simulink model "Copy_of_CM13_2024a_MachE_for_UA_HIL"  (R2024a)
settings: Solver=ode1  StartTime=0.0  StopTime=Inf  FixedStep=0.001  RelTol=1e-3  EnableMultiTasking=on
PreLoadFcn:
  | % if ~length(which('cmcmd')), cmenv; end
PostLoadFcn:
  | if any(exist('dsrtsu_mdlpostloadfcn', 'file') ~= 0), dsrtsu_mdlpostloadfcn('Execute', bdroot); end
InitFcn:
  | , if any(exist('rtifpga_mdlclblib', 'file') ~= 0), rtifpga_mdlclblib('Init', bdroot); end,
  | , if any(exist('dsmpb_private', 'file') ~= 0), dsmpb_private('dsmpb_mdlclblib', 'Init', bdroot); end,
undefined symbols (not defined in the file or in its folder): AccelCmd, ActTqLF_Nm_, ActTqLR_Nm_, ActTqRF_Nm_, ActTqRR_Nm_, BattChargeLimitMaxPwr, BattChargeLimitSocBpts, BattChargeLimitTbl, BattChrgCapcty, BattDischargeLimitSocBpts, BattDischargeLimitTbl, BattDischargeMaxPwr, BattNumCellsParallel, BattNumCellsSeries, BattOpenVoltCapBpts, BattOpenVoltTbl, BattResistSocBpts, BattResistTbl, BattResistTempBpts, BrakeMaxPrs, BrakeMaxTrq, ChassisDistCg2FrontAxle, ChassisDistCg2RearAxle, ChassisVehMass, CltchCmd, CoastDown, DecelCmd, DiffRatio, DiscIntNeverNeededParam, EnvGravCnst, EnvPrs, EnvTemp, FuelSpecificGrav, GearCmd, h, InitStates, lgSw, limitedMCT, MCT, MtrEffSpdBpts, MtrEffTbl, MtrEffTrqBpts, MtrPwrMax, MtrTrqMax, planned_speed, planned_time, pMCT, RealSimPara, ref_speed, Ref_speed, ref_time, Ref_time, rticanmm_blockfcn, rticanmm_initfcn, SteeringCmd, SupvsryCtrlRegenBrkCutOffTbl, SupvsryCtrlRegenSpdBpts, TestScnrioCycleNum, US06, VEH
libraries: simulink x264, VSIGenLib x262, etargetslib x201, dsmpblib x161, CarMaker4SL x142, rtimmsu_dsrtlib x32, vehdynlibtire x24, autolibshared x19, vehdynlibsuspension x14, vehdynlibtirecommon x14, autolibutils x10, VsrLibWheel x8
(part 4 of 47)

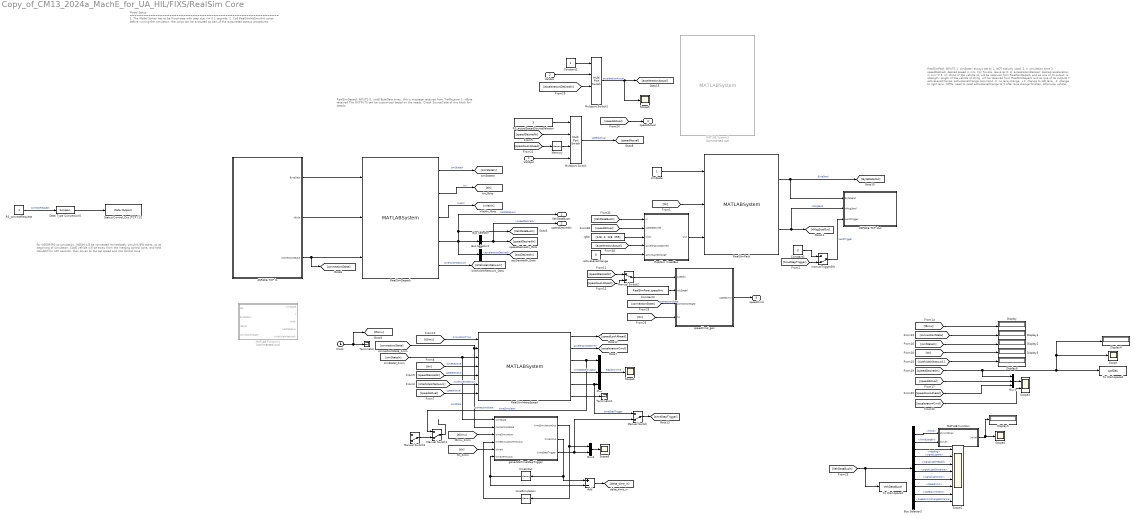
== system Copy_of_CM13_2024a_MachE_for_UA_HIL/FIXS/RealSim Core ==
  note: Model Setup
      | ================================================================
      | 1. The Model Solver has to be Fixed-step with step size <= 0.1 seconds.
      | 2. Call RealSimInitSimulink script before running the simulation. the script can be executed as part of the automated startup procedures.
  note: RealSimDepack
      | INPUTS
      | 0: uint8 ByteData array, this is message received from TrafficLayer
      | 1: nByte received
      |
      | The OUTPUTS can be customized based on the needs. Check SourceCode of this block for details.
  note: RealSimPack
      | INPUTS
      | 1. simState: always set to 1. NOT actively used.
      | 2. t: simulation time
      | 3. speedDesired: desired speed in m/s, For Toyota, leave as 0.
      | 4. accelerationDesired: desired acceleration in m/s^2
      | 5. id: string of the vehicle id, will be received from RealSimDepack and as one of its output.
      | 6. idLength: length of the vehicle id string, will be received from RealSimDepack and as one of its outputs
      | 7: activeLaneChange: activeLaneChange command, 0: no lane change, +1: change to left lane, -1: change to right lane. NOTE: need to reset activeLaneChange to 0 after lane change finishes, otherwise vehicle will keep making lane change. Will receive 0 activeLaneChangeFdbk from RealSimDepack when lane change finishes.
      |
      | NOTE 1: Currently, only speedDesired and/or accelerationDesired can be sent to VISSIM/SUMO. The data format receive and send are the same so other mesage fields of the send data are irrelevant and can be set to empty or zero.
      |
      | NOTE 2: if select both speedDesired and accelerationDesired
      | in config.yaml, then only accelerationDesired will be used
      | to control vehicles in TrafficSimulator. if only one of
      | speedDesired and accelerationDesired selected in
      | config.yaml, then the one selected will be used for
      | control, the other input can be leave as 0.
      |
      | NOTE 3: for VISSIM, speedDesired or accelerationDesired will be the control command 0.2 seconds in the future.
      |
      | OUTPUTS
      | 1.ByteData: bytes vector that will be sent to TrafficSimualtor
      | 2.nMsgSize: size of bytes to be sent
  note: for VISSIM-IPG co-simulation, VISSIM will be connected immediately simulink/IPG starts. so at beginning of simulation, CAVE vehicle will be away from the merging control zone, and held standstill for XXX seconds, then driven to the set speed and into control zone
  VehSpd : Inport
  VehAcc : Inport  Port=2
  Add : Sum  Inputs=+-
  Bus Selector : BusSelector  OutputSignals=speedDesired
  Bus Selector1 : BusSelector  OutputSignals=accelerationDesired
  Bus Selector2 : BusSelector  OutputSignals=linkId,linkIdLength,heading,signalLightId,signalLightHeadId,signalLightDistance,signalLightColor,speedLimit,speedLimitNext,speedLimitChangeDistance
  Clock : Clock
  Constant1 : Constant  Value=0
  Constant2 : Constant
  Constant3 : Constant  Value=RealSimPara.speedInit
  Data Type Conversion5 : DataTypeConversion  OutDataTypeStr=boolean  SaturateOnIntegerOverflow=off  RndMeth=Floor
  Display{,1..6} (7 alike) : Display
  MATLAB Function : MATLAB Function  TreatAsAtomicUnit=on
  MATLAB Function1 : MATLAB Function  Commented=on  TreatAsAtomicUnit=on
  MATLAB System3 : MATLABSystem  Commented=on  System=RealSimPack  VehicleMessageFieldDefInputVec=VehicleMessageFieldDefInputVec  SimulateUsing=Code generation
      mask Type: RealSimPack
      mask Display:
      | disp('RealSimPack');
      | port_label('input',1,'simState');
      | port_label('input',2,'t');
      | port_label('input',3,'VehDataBus');
      | port_label('output',1,'ByteData');
      | port_label('output',2,'nMsgSize');
  Manual Switch : ManualSwitch  CurrentSetting=0
  Manual Switch1 : ManualSwitch  CurrentSetting=0
  Manual Switch2 : ManualSwitch
  Manual Switch3 : ManualSwitch  CurrentSetting=0
  Memory : Memory
  Multiport Switch : MultiPortSwitch  SaturateOnIntegerOverflow=off  InputSameDT=off
  Multiport Switch1 : MultiPortSwitch  SaturateOnIntegerOverflow=off  InputSameDT=off
  Mux : Mux  Inputs=3
  Mux1 : Mux  Inputs=3
  Mux2 : Mux  Inputs=2
  RS_actualSpeedSourceSelector : Constant  Value=3
  RS_connectRequest : Constant
  RealSim CreatBus : Subsystem
  RealSimDepack : MATLABSystem  System=RealSimDepack  OutputBusName=VehDataBus  VehicleMessageFieldDefInputVec=VehicleMessageFieldDefInputVec  SimulateUsing=Code generation
      mask Type: RealSimDepack
      mask Display:
      | disp('RealSimDepack');
      | port_label('input',1,'ByteData');
      | port_label('input',2,'nByte');
      | port_label('input',3,'connectionState');
      | port_label('output',1,'simState');
      | port_label('output',2,'t');
      | port_label('output',3,'nVeh');
      | port_label('output',4,'VehDataBus');
      | port_label('output',5,'isVehicleInNetwork');
  RealSimInterpSpeed : MATLABSystem  System=RealSimInterpSpeed  initialSpeed=RealSimPara.speedInit  speedLookAheadHorizon=RealSimPara.tLookahead  speedUpperBound=30  smoothWindow=RealSimPara.smoothWindow  SimulateUsing=Code generation
      mask Type: RealSimInterpSpeed
      mask Display:
      | disp('RealSimInterpSpeed');
      | port_label('input',1,'simulationTime');
      | port_label('input',2,'connectionState');
      | port_label('input',3,'simState');
      | port_label('input',4,'timeReceive');
      | port_label('input',5,'speedReceive');
      | port_label('input',6,'isVehicleInNetwork');
      | port_label('input',7,'speedActual');
      | port_label('output',1,'speedLookAhead');
      | port_label('output',2,'accelerationDesired');
      | port_label('output',3,'timeSimulator');
      | port_label('output',4,'timeStepSimulator');
      | port_label('output',5,'timeStepTrigger');
      | port_label('output',6,'RealSimDelay');
  RealSimPack : MATLABSystem  System=RealSimPack  VehicleMessageFieldDefInputVec=VehicleMessageFieldDefInputVec  SimulateUsing=Code generation
      mask Type: RealSimPack
      mask Display:
      | disp('RealSimPack');
      | port_label('input',1,'simState');
      | port_label('input',2,'t');
      | port_label('input',3,'VehDataBus');
      | port_label('output',1,'ByteData');
      | port_label('output',2,'nMsgSize');
  Scope{,1,4..6} (5 alike) : Scope
  Scope2 : Scope  NumInputPorts=8
  Scope3 : Scope  NumInputPorts=2
  Status/Control_Out [TCP (1)] : dsmpblib/Data Outport  Priority=-10000
      settings: SourceProductName=dSPACE Model Interface Package for Simulink (MIPS)
  Terminator : Terminator
  Terminator1 : Terminator
  To Workspace1 : ToWorkspace  VariableName=VehDataBusIn  SaveFormat=Timeseries  SampleTime=-1
  To Workspace2 : ToWorkspace  VariableName=spdDes  SaveFormat=Structure With Time  SampleTime=-1
  activeLaneChange : Constant  Value=0
  dSPACE TCP In : Subsystem
  dSPACE TCP Out : Subsystem
  generateTimeStepTrigger : MATLAB Function  TreatAsAtomicUnit=on
  manualTriggerSW : ManualSwitch  CurrentSetting=0
  rgba : Constant  Value=[128, 0, 128, 255]
  simState : Constant
  speedCmd_gen : Subsystem
  timeInOut : Memory
  timeSimulation : Memory
  VehDataBusIn : Outport
  speedDesiredIn : Outport  Port=2
  speedCmd : Outport  Port=3
  speedActual : Outport  Port=4
  wires:
  [speedLookAhead] -> Memory/1
  Bus Selector/1 -> speedDesiredIn/1, [speedDesiredIn]  "<speedDesired>"
  RealSimDepack/1 -> [simStateIn]  "simStateIn"
  Bus Selector2/9 -> Scope2/7  "<speedLimitNext>"
  [tSimu] -> RealSimInterpSpeed/1  "simulationTime"
  RealSimInterpSpeed/4 -> Mux/2  "timeStepSimulator"
  Bus Selector2/1 -> MATLAB Function/1(strUint8Vec)  "<linkId>"
  Bus Selector2/3 -> Scope2/1  "<heading>"
  [tIn] -> RealSimInterpSpeed/4  "timeReceive"
  Bus Selector2/10 -> Scope2/8  "<speedLimitChangeDistance>"
  VehSpd/1 -> Multiport Switch/4
  [speedDesiredIn] -> RealSimInterpSpeed/5  "speedReceive"
  [simStateIn] -> Display2/1
  RealSimDepack/3 -> [nVehIn]  "nVehIn"
  [VehDataBusIn] -> To Workspace1/1, Bus Selector2/1
  [isVehicleInNetwork] -> Display6/1
  Bus Selector2/7 -> Scope2/5  "<signalLightColor>"
  simState/1 -> RealSimPack/1
  RealSimDepack/4 -> Bus Selector1/1, VehDataBusIn/1, [VehDataBusIn], Bus Selector/1  "VehDataBusIn"
  [speedDesiredIn] -> Display4/1, Scope/1, To Workspace2/1, Mux1/1
  RealSimInterpSpeed/2 -> [accelerationCmd]  "accelerationDesired"
  [isVehicleInNetwork] -> RealSimInterpSpeed/6  "isVehicleInNetwork"
  RS_actualSpeedSourceSelector/1 -> Multiport Switch/1
  RealSim CreatBus/1(Out) -> RealSimPack/3
  [accelerationCmd] -> Scope3/2
  Mux/1 -> Scope1/1  "RealSimTime"
  [tIn] -> RealSimPack/2
  Bus Selector2/2 -> MATLAB Function/2(strLen)  "<linkIdLength>"
  Bus Selector2/8 -> Scope2/6  "<speedLimit>"
  [connectionState] -> Display1/1
  RealSimInterpSpeed/5 -> Manual Switch/1, Mux/3  "timeStepTrigger"
  RealSimDepack/5 -> [isVehicleInNetwork]  "isVehicleInNetwork"
  Bus Selector2/5 -> Scope2/3  "<signalLightHeadId>"
  Bus Selector2/6 -> Scope2/4  "<signalLightDistance>"
  RealSimInterpSpeed/6 -> Terminator1/1
  RealSimPack/1 -> dSPACE TCP Out/1(ByteSend), [ByteDataOut]  "ByteSend"
  [tIn] -> Display3/1
  Multiport Switch/1 -> [speedActual]  "speedActual"
  [tSimu] -> Display/1
  [connectionState] -> generateTimeStepTrigger/2(connectionState), RealSimInterpSpeed/2  "connectionState"
  [speedLookAhead] -> Mux1/3
  [speedActual] -> RealSimInterpSpeed/7  "speedActual"
  [simStateIn] -> generateTimeStepTrigger/1(simState), RealSimInterpSpeed/3  "simState"
  RealSimInterpSpeed/1 -> [speedLookAhead]
  Mux1/1 -> Scope3/1
  MATLAB Function/1(intVal) -> Display5/1, Scope4/1
  RealSimPack/2 -> dSPACE TCP Out/2(nMsgSend), [nMsgSizeOut]  "nMsgSend"
  Bus Selector2/4 -> Scope2/2  "<signalLightId>"
  RealSimInterpSpeed/3 -> Mux/1, Manual Switch1/1  "timeSimulator"
  [speedDesiredIn] -> Multiport Switch/2
  [speedActual] -> Mux1/2
  RealSimDepack/2 -> [tIn]  "tIn"
  manualTriggerSW/1 -> dSPACE TCP Out/3(sendTrigger)  "sendTrigger"
  dSPACE TCP In/3(ConnectionState) -> RealSimDepack/3, [connectionState]
  dSPACE TCP In/1(ByteData) -> RealSimDepack/1
  dSPACE TCP In/2(nByte) -> RealSimDepack/2
  Data Type Conversion5/1 -> Status/Control_Out [TCP (1)]/1
  RS_connectRequest/1 -> Data Type Conversion5/1  "connectRequest"
  Memory/1 -> Multiport Switch/3
  Clock/1 -> Terminator/1, [tSimu]
  timeSimulation/1 -> generateTimeStepTrigger/4(timeSimulationPrevious)
  generateTimeStepTrigger/3(timeStepTrigger) -> Manual Switch/2, Mux2/2
  generateTimeStepTrigger/1(timeSimulationOut) -> Mux2/1, timeSimulation/1
  Mux2/1 -> Scope6/1
  Manual Switch/1 -> [timeStepTrigger]
  [timeStepTrigger] -> manualTriggerSW/2
  Constant1/1 -> manualTriggerSW/1
  ? -> Manual Switch3/1
  [speedDesiredIn] -> Manual Switch2/1
  [speedLookAhead] -> Manual Switch2/2
  [speedActual] -> speedActual/1
  Manual Switch2/1 -> speedCmd_gen/1(speedIn)
  Constant3/1 -> speedCmd_gen/2(initSpeed)
  speedCmd_gen/1(speedCmd) -> speedCmd/1
  [connectionState] -> speedCmd_gen/3(connectionState)  "connectionState"
  [tIn] -> speedCmd_gen/4(tIn)
  ? -> Manual Switch3/2
  Manual Switch3/1 -> Manual Switch1/2
  generateTimeStepTrigger/2(timeInOut) -> Add/1, timeInOut/1
  timeInOut/1 -> Add/2, generateTimeStepTrigger/6(timeInPrevious)
  [VehDataBusIn] -> RealSim CreatBus/1(In)
  rgba/1 -> RealSim CreatBus/3(color)
  activeLaneChange/1 -> RealSim CreatBus/5(activeLaneChange)
  [speedActual] -> RealSim CreatBus/2(speedDesired)
  Bus Selector1/1 -> [accDesiredIn]  "<accelerationDesired>"
  [accelerationDesiredIn] -> Multiport Switch1/3
  VehAcc/1 -> Multiport Switch1/2
  Constant2/1 -> Multiport Switch1/1
  Multiport Switch1/1 -> [accelerationActual], Scope5/1  "accelerationActual"
  [accelerationActual] -> RealSim CreatBus/4(accelerationDesired)
  Manual Switch1/1 -> ?
  [tSimu] -> generateTimeStepTrigger/3(timeSimulation)
  [tIn] -> generateTimeStepTrigger/5(timeIn)
  Add/1 -> [delta_time_in]

== system Copy_of_CM13_2024a_MachE_for_UA_HIL/FIXS1/RealSim Core ==
  note: Model Setup
      | ================================================================
      | 1. The Model Solver has to be Fixed-step with step size <= 0.1 seconds.
      | 2. Call RealSimInitSimulink script before running the simulation. the script can be executed as part of the automated startup procedures.
  note: RealSimDepack
      | INPUTS
      | 0: uint8 ByteData array, this is message received from TrafficLayer
      | 1: nByte received
      |
      | The OUTPUTS can be customized based on the needs. Check SourceCode of this block for details.
  note: RealSimPack
      | INPUTS
      | 1. simState: always set to 1. NOT actively used.
      | 2. t: simulation time
      | 3. speedDesired: desired speed in m/s, For Toyota, leave as 0.
      | 4. accelerationDesired: desired acceleration in m/s^2
      | 5. id: string of the vehicle id, will be received from RealSimDepack and as one of its output.
      | 6. idLength: length of the vehicle id string, will be received from RealSimDepack and as one of its outputs
      | 7: activeLaneChange: activeLaneChange command, 0: no lane change, +1: change to left lane, -1: change to right lane. NOTE: need to reset activeLaneChange to 0 after lane change finishes, otherwise vehicle will keep making lane change. Will receive 0 activeLaneChangeFdbk from RealSimDepack when lane change finishes.
      |
      | NOTE 1: Currently, only speedDesired and/or accelerationDesired can be sent to VISSIM/SUMO. The data format receive and send are the same so other mesage fields of the send data are irrelevant and can be set to empty or zero.
      |
      | NOTE 2: if select both speedDesired and accelerationDesired
      | in config.yaml, then only accelerationDesired will be used
      | to control vehicles in TrafficSimulator. if only one of
      | speedDesired and accelerationDesired selected in
      | config.yaml, then the one selected will be used for
      | control, the other input can be leave as 0.
      |
      | NOTE 3: for VISSIM, speedDesired or accelerationDesired will be the control command 0.2 seconds in the future.
      |
      | OUTPUTS
      | 1.ByteData: bytes vector that will be sent to TrafficSimualtor
      | 2.nMsgSize: size of bytes to be sent
  note: for VISSIM-IPG co-simulation, VISSIM will be connected immediately simulink/IPG starts. so at beginning of simulation, CAVE vehicle will be away from the merging control zone, and held standstill for XXX seconds, then driven to the set speed and into control zone
  VehDataBusOut : Inport
  CM_speed : Inport  Port=2
  Bus Selector : BusSelector  OutputSignals=speedDesired
  Bus Selector2 : BusSelector  OutputSignals=linkId,linkIdLength,heading,signalLightId,signalLightHeadId,signalLightDistance,signalLightColor,speedLimit,speedLimitNext,speedLimitChangeDistance
  Clock : Clock
  Constant : Constant
  Constant1 : Constant  Value=0
  Constant3 : Constant  Value=RealSimPara.speedInit
  Data Type Conversion5 : DataTypeConversion  OutDataTypeStr=boolean  SaturateOnIntegerOverflow=off  RndMeth=Floor
  Display{,1..6} (7 alike) : Display
  MATLAB Function : MATLAB Function  TreatAsAtomicUnit=on
  MATLAB Function1 : MATLAB Function  Commented=on  TreatAsAtomicUnit=on
  MATLAB System : MATLABSystem  System=RealSimDepack  OutputBusName=VehDataBus  VehicleMessageFieldDefInputVec=VehicleMessageFieldDefInputVec  SimulateUsing=Code generation
      mask Type: RealSimDepack
      mask Display:
      | disp('RealSimDepack');
      | port_label('input',1,'ByteData');
      | port_label('input',2,'nByte');
      | port_label('input',3,'connectionState');
      | port_label('output',1,'simState');
      | port_label('output',2,'t');
      | port_label('output',3,'nVeh');
      | port_label('output',4,'VehDataBus');
      | port_label('output',5,'isVehicleInNetwork');
  MATLAB System1 : MATLABSystem  System=RealSimPack  VehicleMessageFieldDefInputVec=VehicleMessageFieldDefInputVec  SimulateUsing=Code generation
      mask Type: RealSimPack
      mask Display:
      | disp('RealSimPack');
      | port_label('input',1,'simState');
      | port_label('input',2,'t');
      | port_label('input',3,'VehDataBus');
      | port_label('output',1,'ByteData');
      | port_label('output',2,'nMsgSize');
  Manual Switch : ManualSwitch  CurrentSetting=0
  Manual Switch1 : ManualSwitch  CurrentSetting=0
  Manual Switch2 : ManualSwitch
  Manual Switch3 : ManualSwitch  CurrentSetting=0
  Memory : Memory
  Memory1 : Memory
  Memory2 : Memory
  Multiport Switch : MultiPortSwitch  SaturateOnIntegerOverflow=off  InputSameDT=off
  Mux : Mux  Inputs=3
  Mux1 : Mux  Inputs=3
  Mux2 : Mux  Inputs=2
  RS_actualSpeedSourceSelector : Constant  Value=3
  RS_connectRequest : Constant  Value=0
  Read CM Dict7 : CarMaker4SL/Read CM Dict  xname=SC.State  xsync=off  xstime=Continuous
  RealSimInterpSpeed : MATLABSystem  System=RealSimInterpSpeed  initialSpeed=RealSimPara.speedInit  speedLookAheadHorizon=RealSimPara.tLookahead  speedUpperBound=30  smoothWindow=RealSimPara.smoothWindow  SimulateUsing=Code generation
      mask Type: RealSimInterpSpeed
      mask Display:
      | disp('RealSimInterpSpeed');
      | port_label('input',1,'simulationTime');
      | port_label('input',2,'connectionState');
      | port_label('input',3,'simState');
      | port_label('input',4,'timeReceive');
      | port_label('input',5,'speedReceive');
      | port_label('input',6,'isVehicleInNetwork');
      | port_label('input',7,'speedActual');
      | port_label('output',1,'speedLookAhead');
      | port_label('output',2,'accelerationDesired');
      | port_label('output',3,'timeSimulator');
      | port_label('output',4,'timeStepSimulator');
      | port_label('output',5,'timeStepTrigger');
      | port_label('output',6,'RealSimDelay');
  Scope{,1,4,6} (4 alike) : Scope
  Scope2 : Scope  NumInputPorts=8
  Scope3 : Scope  NumInputPorts=2
  Status/Control_Out [TCP (1)] : dsmpblib/Data Outport  Priority=-10000
      settings: SourceProductName=dSPACE Model Interface Package for Simulink (MIPS)
  Subsystem : Subsystem
  Switch : Switch  Threshold=6  SaturateOnIntegerOverflow=off  InputSameDT=off
  Terminator : Terminator
  Terminator1 : Terminator
  To Workspace1 : ToWorkspace  VariableName=VehDataBusIn  SaveFormat=Timeseries  SampleTime=-1
  To Workspace2 : ToWorkspace  VariableName=spdDes  SaveFormat=Structure With Time  SampleTime=-1
  dSPACE TCP In : Subsystem
  dSPACE TCP Out : Subsystem
  generateTimeStepTrigger : MATLAB Function  TreatAsAtomicUnit=on
  manualTriggerSW : ManualSwitch  CurrentSetting=0
  simState : Constant
  VehDataBusIn : Outport
  speedDesiredIn : Outport  Port=2
  speedCmd : Outport  Port=3
  speedActual : Outport  Port=4
  wires:
  [speedLookAhead] -> Memory/1
  Bus Selector/1 -> speedDesiredIn/1, [speedDesiredIn]  "<speedDesired>"
  MATLAB System/1 -> [simStateIn]  "simStateIn"
  Bus Selector2/9 -> Scope2/7  "<speedLimitNext>"
  [tSimu] -> RealSimInterpSpeed/1  "simulationTime"
  RealSimInterpSpeed/4 -> Mux/2  "timeStepSimulator"
  Bus Selector2/1 -> MATLAB Function/1(strUint8Vec)  "<linkId>"
  Bus Selector2/3 -> Scope2/1  "<heading>"
  [tIn] -> RealSimInterpSpeed/4  "timeReceive"
  Bus Selector2/10 -> Scope2/8  "<speedLimitChangeDistance>"
  CM_speed/1 -> Multiport Switch/4
  [speedDesiredIn] -> RealSimInterpSpeed/5  "speedReceive"
  [simStateIn] -> Display2/1
  MATLAB System/3 -> [nVehIn]  "nVehIn"
  [VehDataBusIn] -> To Workspace1/1, Bus Selector2/1
  [isVehicleInNetwork] -> Display6/1
  Bus Selector2/7 -> Scope2/5  "<signalLightColor>"
  simState/1 -> MATLAB System1/1
  MATLAB System/4 -> VehDataBusIn/1, [VehDataBusIn], Bus Selector/1  "VehDataBusIn"
  [speedDesiredIn] -> Display4/1, Scope/1, To Workspace2/1, Mux1/1
  RealSimInterpSpeed/2 -> [accelerationCmd]  "accelerationDesired"
  [isVehicleInNetwork] -> RealSimInterpSpeed/6  "isVehicleInNetwork"
  RS_actualSpeedSourceSelector/1 -> Multiport Switch/1
  VehDataBusOut/1 -> MATLAB System1/3
  [accelerationCmd] -> Scope3/2
  Mux/1 -> Scope1/1  "RealSimTime"
  [tIn] -> MATLAB System1/2
  Bus Selector2/2 -> MATLAB Function/2(strLen)  "<linkIdLength>"
  Bus Selector2/8 -> Scope2/6  "<speedLimit>"
  [connectionState] -> Display1/1
  RealSimInterpSpeed/5 -> Manual Switch/1, Mux/3  "timeStepTrigger"
  MATLAB System/5 -> [isVehicleInNetwork]  "isVehicleInNetwork"
  Bus Selector2/5 -> Scope2/3  "<signalLightHeadId>"
  Bus Selector2/6 -> Scope2/4  "<signalLightDistance>"
  RealSimInterpSpeed/6 -> Terminator1/1
  MATLAB System1/1 -> dSPACE TCP Out/1(ByteSend), [ByteDataOut]  "ByteSend"
  [tIn] -> Display3/1
  Multiport Switch/1 -> [speedActual]  "speedActual"
  [tSimu] -> Display/1
  [connectionState] -> generateTimeStepTrigger/2(connectionState), RealSimInterpSpeed/2  "connectionState"
  [speedLookAhead] -> Mux1/3
  [speedActual] -> RealSimInterpSpeed/7  "speedActual"
  [simStateIn] -> generateTimeStepTrigger/1(simState), RealSimInterpSpeed/3  "simState"
  RealSimInterpSpeed/1 -> [speedLookAhead]
  Mux1/1 -> Scope3/1
  MATLAB Function/1(intVal) -> Scope4/1, Display5/1
  MATLAB System1/2 -> dSPACE TCP Out/2(nMsgSend), [nMsgSizeOut]  "nMsgSend"
  Bus Selector2/4 -> Scope2/2  "<signalLightId>"
  RealSimInterpSpeed/3 -> Mux/1, Manual Switch1/1  "timeSimulator"
  [speedDesiredIn] -> Multiport Switch/2
  [speedActual] -> Mux1/2
  MATLAB System/2 -> [tIn]  "tIn"
  manualTriggerSW/1 -> dSPACE TCP Out/3(sendTrigger)
  dSPACE TCP In/3(ConnectionState) -> [connectionState], MATLAB System/3
  dSPACE TCP In/1(ByteData) -> MATLAB System/1
  dSPACE TCP In/2(nByte) -> MATLAB System/2
  Data Type Conversion5/1 -> Status/Control_Out [TCP (1)]/1
  Switch/1 -> Data Type Conversion5/1  "connectRequest"
  Memory/1 -> Multiport Switch/3
  Clock/1 -> Terminator/1, [tSimu]
  RS_connectRequest/1 -> Switch/3
  Read CM Dict7/1 -> Switch/2  "SimCore_State"
  Constant/1 -> Switch/1
  Memory1/1 -> generateTimeStepTrigger/4(timeSimulationPrevious)
  generateTimeStepTrigger/3(timeStepTrigger) -> Manual Switch/2, Mux2/2
  generateTimeStepTrigger/1(timeSimulationOut) -> Memory1/1, Mux2/1
  Mux2/1 -> Scope6/1
  Manual Switch/1 -> [timeStepTrigger]
  [timeStepTrigger] -> manualTriggerSW/2
  Constant1/1 -> manualTriggerSW/1
  Manual Switch1/1 -> generateTimeStepTrigger/3(timeSimulation)
  [tIn] -> generateTimeStepTrigger/5(timeIn), Manual Switch3/1
  [speedDesiredIn] -> Manual Switch2/1
  [speedLookAhead] -> Manual Switch2/2
  [speedActual] -> speedActual/1
  Manual Switch2/1 -> Subsystem/1(speedIn)
  Constant3/1 -> Subsystem/2(initSpeed)
  Subsystem/1(speedCmd) -> speedCmd/1
  [connectionState] -> Subsystem/3(connectionState)  "connectionState"
  [tIn] -> Subsystem/4(tIn)
  [tSimu] -> Manual Switch3/2
  Manual Switch3/1 -> Manual Switch1/2
  generateTimeStepTrigger/2(timeInOut) -> Memory2/1
  Memory2/1 -> generateTimeStepTrigger/6(timeInPrevious)

== system Copy_of_CM13_2024a_MachE_for_UA_HIL/FIXS1/RealSim Translate CM Signal to Bus as Feedback to SUMO//VISSIM ==
  VehDataBusIn : Inport
  speedActual : Inport  Port=2
  Constant : Constant  Value=[255,0,0,255]
  MATLAB Function : MATLAB Function  TreatAsAtomicUnit=on
  Read CM Dict : CarMaker4SL/Read CM Dict  xname=Vhcl.Fr1.x  xsync=off  xstime=Continuous
  Read CM Dict1 : CarMaker4SL/Read CM Dict  xname=Vhcl.PoI.x  xsync=off  xstime=Continuous
  Read CM Dict2 : CarMaker4SL/Read CM Dict  xname=Vhcl.v  xsync=off  xstime=Continuous
  Read CM Dict3 : CarMaker4SL/Read CM Dict  xname=Vhcl.Yaw  xsync=off  xstime=Continuous
  Read CM Dict4 : CarMaker4SL/Read CM Dict  xname=Vhcl.Fr1.y  xsync=off  xstime=Continuous
  Read CM Dict5 : CarMaker4SL/Read CM Dict  xname=Vhcl.Fr1.z  xsync=off  xstime=Continuous
  Read CM Dict6 : CarMaker4SL/Read CM Dict  xname=Vhcl.PoI.y  xsync=off  xstime=Continuous
  Read CM Dict7 : CarMaker4SL/Read CM Dict  xname=Vhcl.PoI.z  xsync=off  xstime=Continuous
  RealSim CreatBus : Subsystem
  RealSim CreatBus2 : Subsystem  Commented=on
  Terminator{1..4} (4 alike) : Terminator
  accelerationDesired : Constant  Value=0
  activeLaneChange : Constant  Value=0
  VehDataBusOut : Outport
  CM_speed : Outport  Port=2
  wires:
  Read CM Dict6/1 -> MATLAB Function/2(CM_POI_Y)
  speedActual/1 -> RealSim CreatBus/2(speedDesired)
  MATLAB Function/4(heading) -> Terminator3/1
  Read CM Dict2/1 -> CM_speed/1, MATLAB Function/9(CM_speed)
  Read CM Dict4/1 -> MATLAB Function/5(CM_Fr1_Y)
  MATLAB Function/2(positionY) -> Terminator1/1
  MATLAB Function/1(positionX) -> RealSim CreatBus/6(positionX)
  Read CM Dict/1 -> MATLAB Function/4(CM_Fr1_X)
  MATLAB Function/3(positionZ) -> Terminator2/1
  Read CM Dict7/1 -> MATLAB Function/3(CM_POI_Z)
  MATLAB Function/5(color) -> RealSim CreatBus/3(color)
  Constant/1 -> MATLAB Function/8(color_rgba)
  Read CM Dict5/1 -> MATLAB Function/6(CM_Fr1_Z)
  Read CM Dict1/1 -> MATLAB Function/1(CM_POI_X)
  Read CM Dict3/1 -> MATLAB Function/7(CM_yaw)
  VehDataBusIn/1 -> RealSim CreatBus/1(VehDataBusIn)
  RealSim CreatBus/1(Out) -> VehDataBusOut/1
  activeLaneChange/1 -> RealSim CreatBus/5(activeLaneChange)
  accelerationDesired/1 -> RealSim CreatBus/4(accelerationDesired)
  MATLAB Function/6(speedDesired) -> Terminator4/1

== system Copy_of_CM13_2024a_MachE_for_UA_HIL/RealSim1/FromRealSim ==
  note: RealSimDepack
      | INPUTS
      | 0: uint8 ByteData array, this is message received from TrafficLayer
      | 1: nByte received
      |
      | The OUTPUTS can be customized based on the needs. Check SourceCode of this block for details.
  note: RealSimSocket
      | PARAMETERS:
      | 0: ip address of the RealSim TrafficLayer
      | 1: port to RealSim TrafficLayer
      | 2: enable log or not, disable for performance
      | INPUT:
      | 0: simulation time
      | 1: dt, frequency to receive and send to Traffic Simulator, has to be 0.1 for now, DO NOT change
      | 2: enable connection, 1: enable, 0: close. NOT currently used.
      | 3: ByteData to send
      | 4: nMsgSize
      |
      | OUTPUT:
      | 0: uint8 ByteData array
      | 1: nByte received
      | 2: connection flag, 1: connected to TrafficSimulator, 0: not connected
  tSimu : Inport
  dt : Inport  Port=2
  enableConnection : Inport  Port=3
  byteDataOut : Inport  Port=4
  nMsgSizeOut : Inport  Port=5
  Data Type Conversion1 : DataTypeConversion  OutDataTypeStr=uint8  SaturateOnIntegerOverflow=off  RndMeth=Floor
  Data Type Conversion2 : DataTypeConversion  OutDataTypeStr=boolean  SaturateOnIntegerOverflow=off  RndMeth=Floor
  Data Type Conversion3 : DataTypeConversion  OutDataTypeStr=double  SaturateOnIntegerOverflow=off  RndMeth=Floor
  Display8 : Display
  MATLAB System : MATLABSystem  System=RealSimDepack  OutputBusName=VehDataBus  VehicleMessageFieldDefInputVec=VehicleMessageFieldDefInputVec  SimulateUsing=Interpreted execution
      mask Type: RealSimDepack
      mask Display:
      | disp('RealSimDepack');
      | port_label('input',1,'ByteData');
      | port_label('input',2,'nByte');
      | port_label('input',3,'connectionState');
      | port_label('output',1,'simState');
      | port_label('output',2,'t');
      | port_label('output',3,'nVeh');
      | port_label('output',4,'VehDataBus');
      | port_label('output',5,'isVehicleInNetwork');
  S-Function : S-Function  FunctionName=RealSimSocket  Parameters=TrafficLayerIP, TrafficLayerPort, 1  SFunctionDeploymentMode=off  EnableBusSupport=off
  Signal Specification : SignalSpecification  Dimensions=[200 1]
  simState : Outport
  t : Outport  Port=2
  nVeh : Outport  Port=3
  VehDataBus : Outport  Port=4
  isVehicleInNetwork : Outport  Port=5
  connectionState : Outport  Port=6
  wires:
  Data Type Conversion3/1 -> MATLAB System/3, [connectionState], connectionState/1
  enableConnection/1 -> Data Type Conversion2/1
  dt/1 -> S-Function/2
  tSimu/1 -> S-Function/1
  MATLAB System/5 -> isVehicleInNetwork/1
  MATLAB System/3 -> nVeh/1
  MATLAB System/1 -> simState/1
  MATLAB System/4 -> VehDataBus/1
  S-Function/1 -> Data Type Conversion1/1
  Data Type Conversion2/1 -> S-Function/3
  Signal Specification/1 -> S-Function/4
  S-Function/2 -> MATLAB System/2, Display8/1
  Data Type Conversion1/1 -> MATLAB System/1
  byteDataOut/1 -> Signal Specification/1
  MATLAB System/2 -> t/1
  S-Function/3 -> Data Type Conversion3/1
  nMsgSizeOut/1 -> S-Function/5

== system Copy_of_CM13_2024a_MachE_for_UA_HIL/RealSim1/SwitchVehicleSpeed ==
  speedIn : Inport
  initialSpeed : Inport  Port=2
  Clock : Clock
  Switch : Switch  Criteria=u2 > Threshold  Threshold=RealSimPara.warmupTime  SaturateOnIntegerOverflow=off  InputSameDT=off
  speedCmd : Outport
  wires:
  initialSpeed/1 -> Switch/3
  Clock/1 -> Switch/2
  speedIn/1 -> Switch/1
  Switch/1 -> speedCmd/1

== system Copy_of_CM13_2024a_MachE_for_UA_HIL/RealSim1/ToRealSim ==
  note: RealSimPack
      | INPUTS
      | 1. simState: always set to 1. NOT actively used.
      | 2. t: simulation time
      | 3. speedDesired: desired speed in m/s, For Toyota, leave as 0.
      | 4. accelerationDesired: desired acceleration in m/s^2
      | 5. id: string of the vehicle id, will be received from RealSimDepack and as one of its output.
      | 6. idLength: length of the vehicle id string, will be received from RealSimDepack and as one of its outputs
      | 7: activeLaneChange: activeLaneChange command, 0: no lane change, +1: change to left lane, -1: change to right lane. NOTE: need to reset activeLaneChange to 0 after lane change finishes, otherwise vehicle will keep making lane change. Will receive 0 activeLaneChangeFdbk from RealSimDepack when lane change finishes.
      |
      | NOTE 1: Currently, only speedDesired and/or accelerationDesired can be sent to VISSIM/SUMO. The data format receive and send are the same so other mesage fields of the send data are irrelevant and can be set to empty or zero.
      |
      | NOTE 2: if select both speedDesired and accelerationDesired
      | in config.yaml, then only accelerationDesired will be used
      | to control vehicles in TrafficSimulator. if only one of
      | speedDesired and accelerationDesired selected in
      | config.yaml, then the one selected will be used for
      | control, the other input can be leave as 0.
      |
      | NOTE 3: for VISSIM, speedDesired or accelerationDesired will be the control command 0.2 seconds in the future.
      |
      | OUTPUTS
      | 1.ByteData: bytes vector that will be sent to TrafficSimualtor
      | 2.nMsgSize: size of bytes to be sent
  In1 : Inport
  In2 : Inport  Port=2
  speedDesired : Inport  Port=3
  accelerationDesired : Inport  Port=4
  MATLAB System1 : MATLABSystem  System=RealSimPack  VehicleMessageFieldDefInputVec=VehicleMessageFieldDefInputVec  SimulateUsing=Code generation
      mask Type: RealSimPack
      mask Display:
      | disp('RealSimPack');
      | port_label('input',1,'simState');
      | port_label('input',2,'t');
      | port_label('input',3,'VehDataBus');
      | port_label('output',1,'ByteData');
      | port_label('output',2,'nMsgSize');
  RealSim CreatBus : Subsystem
  activeLaneChange : Constant  Value=0
  rgba : Constant  Value=[255,0,0,255]
  simState : Constant
  ByteSend : Outport
  nMsgSend : Outport  Port=2
  wires:
  In2/1 -> RealSim CreatBus/1(In)
  MATLAB System1/1 -> ByteSend/1  "ByteSend"
  activeLaneChange/1 -> RealSim CreatBus/5(activeLaneChange)
  RealSim CreatBus/1(Out) -> MATLAB System1/3
  accelerationDesired/1 -> RealSim CreatBus/4(accelerationDesired)
  simState/1 -> MATLAB System1/1
  In1/1 -> MATLAB System1/2
  speedDesired/1 -> RealSim CreatBus/2(speedDesired)
  MATLAB System1/2 -> nMsgSend/1  "nMsgSend"
  rgba/1 -> RealSim CreatBus/3(color)

== system Copy_of_CM13_2024a_MachE_for_UA_HIL/RealSim2/FromRealSim ==
  note: RealSimSocket
      | PARAMETERS:
      | 0: ip address of the RealSim TrafficLayer
      | 1: port to RealSim TrafficLayer
      | 2: enable log or not, disable for performance
      | INPUT:
      | 0: simulation time
      | 1: dt, frequency to receive and send to Traffic Simulator, has to be 0.1 for now, DO NOT change
      | 2: enable connection, 1: enable, 0: close. NOT currently used.
      | 3: ByteData to send
      | 4: nMsgSize
      |
      | OUTPUT:
      | 0: uint8 ByteData array
      | 1: nByte received
      | 2: connection flag, 1: connected to TrafficSimulator, 0: not connected
  note: RealSimDepack
      | INPUTS
      | 0: uint8 ByteData array, this is message received from TrafficLayer
      | 1: nByte received
      |
      | The OUTPUTS can be customized based on the needs. Check SourceCode of this block for details.
  tSimu : Inport
  dt : Inport  Port=2
  enableConnection : Inport  Port=3
  byteDataOut : Inport  Port=4
  nMsgSizeOut : Inport  Port=5
  Data Type Conversion1 : DataTypeConversion  OutDataTypeStr=uint8  SaturateOnIntegerOverflow=off  RndMeth=Floor
  Data Type Conversion2 : DataTypeConversion  OutDataTypeStr=boolean  SaturateOnIntegerOverflow=off  RndMeth=Floor
  Data Type Conversion3 : DataTypeConversion  OutDataTypeStr=double  SaturateOnIntegerOverflow=off  RndMeth=Floor
  Display8 : Display
  MATLAB System : MATLABSystem  System=RealSimDepack  OutputBusName=VehDataBus  VehicleMessageFieldDefInputVec=VehicleMessageFieldDefInputVec  SimulateUsing=Interpreted execution
      mask Type: RealSimDepack
      mask Display:
      | disp('RealSimDepack');
      | port_label('input',1,'ByteData');
      | port_label('input',2,'nByte');
      | port_label('input',3,'connectionState');
      | port_label('output',1,'simState');
      | port_label('output',2,'t');
      | port_label('output',3,'nVeh');
      | port_label('output',4,'VehDataBus');
      | port_label('output',5,'isVehicleInNetwork');
  S-Function : S-Function  FunctionName=RealSimSocket  Parameters=TrafficLayerIP, TrafficLayerPort, 1  SFunctionDeploymentMode=off  EnableBusSupport=off
  Signal Specification : SignalSpecification  Dimensions=[200 1]
  simState : Outport
  t : Outport  Port=2
  nVeh : Outport  Port=3
  VehDataBus : Outport  Port=4
  isVehicleInNetwork : Outport  Port=5
  connectionState : Outport  Port=6
  wires:
  nMsgSizeOut/1 -> S-Function/5
  S-Function/3 -> Data Type Conversion3/1
  MATLAB System/2 -> t/1
  byteDataOut/1 -> Signal Specification/1
  Data Type Conversion1/1 -> MATLAB System/1
  S-Function/2 -> Display8/1, MATLAB System/2
  Signal Specification/1 -> S-Function/4
  Data Type Conversion2/1 -> S-Function/3
  S-Function/1 -> Data Type Conversion1/1
  MATLAB System/4 -> VehDataBus/1
  MATLAB System/1 -> simState/1
  MATLAB System/3 -> nVeh/1
  MATLAB System/5 -> isVehicleInNetwork/1
  tSimu/1 -> S-Function/1
  dt/1 -> S-Function/2
  enableConnection/1 -> Data Type Conversion2/1
  Data Type Conversion3/1 -> connectionState/1, [connectionState], MATLAB System/3

== system Copy_of_CM13_2024a_MachE_for_UA_HIL/RealSim2/SwitchVehicleSpeed ==
  speedIn : Inport
  initialSpeed : Inport  Port=2
  Clock : Clock
  Switch : Switch  Criteria=u2 > Threshold  Threshold=RealSimPara.warmupTime  SaturateOnIntegerOverflow=off  InputSameDT=off
  speedCmd : Outport
  wires:
  Switch/1 -> speedCmd/1
  speedIn/1 -> Switch/1
  Clock/1 -> Switch/2
  initialSpeed/1 -> Switch/3

== system Copy_of_CM13_2024a_MachE_for_UA_HIL/RealSim2/ToRealSim ==
  note: RealSimPack
      | INPUTS
      | 1. simState: always set to 1. NOT actively used.
      | 2. t: simulation time
      | 3. speedDesired: desired speed in m/s, For Toyota, leave as 0.
      | 4. accelerationDesired: desired acceleration in m/s^2
      | 5. id: string of the vehicle id, will be received from RealSimDepack and as one of its output.
      | 6. idLength: length of the vehicle id string, will be received from RealSimDepack and as one of its outputs
      | 7: activeLaneChange: activeLaneChange command, 0: no lane change, +1: change to left lane, -1: change to right lane. NOTE: need to reset activeLaneChange to 0 after lane change finishes, otherwise vehicle will keep making lane change. Will receive 0 activeLaneChangeFdbk from RealSimDepack when lane change finishes.
      |
      | NOTE 1: Currently, only speedDesired and/or accelerationDesired can be sent to VISSIM/SUMO. The data format receive and send are the same so other mesage fields of the send data are irrelevant and can be set to empty or zero.
      |
      | NOTE 2: if select both speedDesired and accelerationDesired
      | in config.yaml, then only accelerationDesired will be used
      | to control vehicles in TrafficSimulator. if only one of
      | speedDesired and accelerationDesired selected in
      | config.yaml, then the one selected will be used for
      | control, the other input can be leave as 0.
      |
      | NOTE 3: for VISSIM, speedDesired or accelerationDesired will be the control command 0.2 seconds in the future.
      |
      | OUTPUTS
      | 1.ByteData: bytes vector that will be sent to TrafficSimualtor
      | 2.nMsgSize: size of bytes to be sent
  In1 : Inport
  In2 : Inport  Port=2
  speedDesired : Inport  Port=3
  accelerationDesired : Inport  Port=4
  MATLAB System1 : MATLABSystem  System=RealSimPack  VehicleMessageFieldDefInputVec=VehicleMessageFieldDefInputVec  SimulateUsing=Code generation
      mask Type: RealSimPack
      mask Display:
      | disp('RealSimPack');
      | port_label('input',1,'simState');
      | port_label('input',2,'t');
      | port_label('input',3,'VehDataBus');
      | port_label('output',1,'ByteData');
      | port_label('output',2,'nMsgSize');
  RealSim CreatBus : Subsystem
  activeLaneChange : Constant  Value=0
  rgba : Constant  Value=[255,0,0,255]
  simState : Constant
  ByteSend : Outport
  nMsgSend : Outport  Port=2
  wires:
  rgba/1 -> RealSim CreatBus/3(color)
  MATLAB System1/2 -> nMsgSend/1  "nMsgSend"
  speedDesired/1 -> RealSim CreatBus/2(speedDesired)
  In1/1 -> MATLAB System1/2
  simState/1 -> MATLAB System1/1
  accelerationDesired/1 -> RealSim CreatBus/4(accelerationDesired)
  RealSim CreatBus/1(Out) -> MATLAB System1/3
  activeLaneChange/1 -> RealSim CreatBus/5(activeLaneChange)
  MATLAB System1/1 -> ByteSend/1  "ByteSend"
  In2/1 -> RealSim CreatBus/1(In)

== system Copy_of_CM13_2024a_MachE_for_UA_HIL/Vehicle Under Test2/Environment ==
  Grade : Inport
  Friction : Constant  Value=ones(4,1).*1
  Ground Feedback : Subsystem  Variant=on  VariantControlMode=label  LabelModeActiveChoice=0
  Ground Z Level : Constant  Value=zeros(4,1)
  Subsystem : Subsystem
  Subsystem1 : Subsystem
      mask Display: disp('')
  Env : Outport
  wires:
  Subsystem/3(WindVel) -> Subsystem1/3(WindVel)
  Subsystem/2(EnvTemp) -> Subsystem1/2(EnvTemp)
  Subsystem/4(RoadGrade) -> Subsystem1/4(RoadGrade)
  Subsystem/1(EnvPrs) -> Subsystem1/1(EnvPrs)
  Subsystem1/1(Env) -> Env/1
  Friction/1 -> Ground Feedback/1(Friction)
  Ground Feedback/1(Ground) -> Subsystem1/5(GroundBus)  "Gnd"
  Ground Z Level/1 -> Ground Feedback/2(Ground Z Level)
  Grade/1 -> Subsystem/1(Grade)

== system Copy_of_CM13_2024a_MachE_for_UA_HIL/Vehicle Under Test2/Monitor ==
  Monitor : Inport
  Calculate Fuel MPG : Subsystem  Commented=on
  Calculate Powertrain Energy : Subsystem
  Terminator : Terminator
  Terminator3 : Terminator
  wires:
  Calculate Fuel MPG/1(FuelEconMPG) -> Terminator/1  "FuelEconMpg"
  Monitor/1 -> Calculate Powertrain Energy/1(Monitor), Calculate Fuel MPG/1(Monitor)
  Calculate Powertrain Energy/1(TransEnrgyOutkWh) -> Terminator3/1  "DiffEnrgyInkWh"

== system Copy_of_CM13_2024a_MachE_for_UA_HIL/Vehicle Under Test2/Performance Calculations ==
  VehSpd : Inport
  BattPwr : Inport  Port=2
  Divide : Product  Inputs=*/
  Divide1 : Product  Inputs=*/
  Divide2 : Product  Inputs=*/
  Integrator : Integrator
  Integrator1 : Integrator
  L/100 Km Calc : Product  Inputs=/*
  Product : Product
  Rate Transition3 : RateTransition  Deterministic=off
  Saturation : Saturate  UpperLimit=Inf  LowerLimit=0.001
  Saturation1 : Saturate  UpperLimit=Inf  LowerLimit=1e-3
  Sqrt : Sqrt
  US EPA kwh/USgal equivalent : Constant  Value=33.7
  US MPG Calc : Product  Inputs=*/
  m to 100Km : Gain  Gain=1/1000/100
  m to mile : Gain  Gain=0.000621371
  m^3 per gal : Gain  Gain=0.00378541
  m^3 to L : Gain  Gain=1000
  m^3 to US Gal : Gain  Gain=264.172
  s per h : Constant  Value=3600
  w per kw : Constant  Value=1000
  US MPG : Outport  VectorParamsAs1DForOutWhenUnconnected=off
  L/100Km : Outport  Port=2  VectorParamsAs1DForOutWhenUnconnected=off
  wires:
  VehSpd/1 -> Product/1, Product/2
  Product/1 -> Sqrt/1
  Sqrt/1 -> Integrator/1
  BattPwr/1 -> Divide/1
  US EPA kwh/USgal equivalent/1 -> Divide2/2
  m^3 per gal/1 -> Integrator1/1
  Divide1/1 -> m^3 per gal/1
  s per h/1 -> Divide1/2
  Divide2/1 -> Divide1/1
  Divide/1 -> Divide2/1
  w per kw/1 -> Divide/2
  Rate Transition3/1 -> US MPG/1  "US MPG"
  Saturation1/1 -> US MPG Calc/2
  US MPG Calc/1 -> Rate Transition3/1
  L/100 Km Calc/1 -> L/100Km/1  "L/100Km"
  m to 100Km/1 -> Saturation/1
  Saturation/1 -> L/100 Km Calc/1
  Integrator1/1 -> m^3 to L/1, m^3 to US Gal/1
  m to mile/1 -> US MPG Calc/1
  Integrator/1 -> m to 100Km/1, m to mile/1
  m^3 to L/1 -> L/100 Km Calc/2
  m^3 to US Gal/1 -> Saturation1/1

== system Copy_of_CM13_2024a_MachE_for_UA_HIL/Vehicle Under Test2/Vehicle ==
  note: With tire radius correction of 1.14
  note: NOT USED
  note: Vehicle simulation type:
      | 0- Simulink offline model
      | 1- Rototest HIL model
  note: NOT USED
  Env : Inport
  Driver : Inport  Port=2
  CarCmd : Inport  Port=3
  Abs : Abs  Commented=on  SaturateOnIntegerOverflow=off
  Actuation and Outputs : Subsystem  Commented=on
  AxT : Scope
  AxT2 : Scope  Commented=on
  Battery : Subsystem
  Bus Creator : BusCreator  Inputs=6
  Bus Selector : BusSelector  OutputSignals=Omega
  Bus Selector1 : BusSelector  Commented=on  OutputSignals=BRAKE_LAMP_BOOL_CAN,STEERING_ANGLE_DEG_CAN
  Bus Selector2 : BusSelector  Commented=on  OutputSignals=CarTrqT2W,VehSpd,Fx
  Bus Selector3 : BusSelector  Commented=on  OutputSignals=PT IF WFL rotv,PT IF WFR rotv,PT IF WRL rotv,PT IF WRR rotv
  Constant : Constant  Commented=on  Value=0  SampleTime=-1
  Data Type Conversion : DataTypeConversion  Commented=on  SaturateOnIntegerOverflow=off  RndMeth=Floor
  Data Type Conversion1 : DataTypeConversion  Commented=on  SaturateOnIntegerOverflow=off  RndMeth=Floor
  DriveCycle_trigger : Constant  Commented=on  Value=0
  Driver and Drive Cycle : Subsystem  Commented=on  TreatAsAtomicUnit=on
  From CAN : Subsystem  Commented=on
  From10 : From  Commented=on  GotoTag=VehSpdKph
  From7 : From  Commented=on  GotoTag=RototestInput  TagVisibility=global
  From8 : From  Commented=on  GotoTag=vehSpeedSim  TagVisibility=global
  Front Wheel Drive : Subsystem  Variant=on  VariantControlMode=label  VariantControl=1  LabelModeActiveChoice=Choice
  Gain : Gain  Commented=on  Gain=3.6
  Gain1 : Gain  Commented=on  Gain=3.6*1.1414
  Goto10 : Goto  Commented=on  GotoTag=VehSpdKph
  Goto6 : Goto  Commented=on  GotoTag=RototestInput  TagVisibility=global
  Goto7 : Goto  Commented=on  GotoTag=BrakePressedCAN
  Goto8 : Goto  Commented=on  GotoTag=SteeringCAN
  Goto9 : Goto  Commented=on  GotoTag=OmegaRoto
  Motor : Subsystem
  MtT : Scope
  MtT1 : Scope
  Multiport Switch : MultiPortSwitch  DataPortOrder=Zero-based contiguous  Inputs=2  zeroidx=on  SaturateOnIntegerOverflow=off  InputSameDT=off
  "Powertrain Supervisory Controller " : Subsystem  AncestorBlock=LibPtSupervisoryCtrl/Powertrain Supervisory Controller
  "Rototest UDP RX ExternalMode  " : Subsystem  Commented=on
  "Rototest UDP TX ExternalMode  " : Subsystem  Commented=on
  Rototest and ORNL Interface : Subsystem  Commented=on
  SUMO_speed_level : Constant  Commented=on  Value=0
  Scope : Scope
  Switch : Switch  Commented=on  Threshold=0.1  SaturateOnIntegerOverflow=off  InputSameDT=off
  Terminator{,1..4} (5 alike) : Terminator  Commented=on
  To Workspace1 : ToWorkspace  Commented=on  VariableName=rotoOmega1  SampleTime=-1
      settings: Save2DSignal=2-D array (concatenate along first dimension)
  To Workspace2 : ToWorkspace  Commented=on  VariableName=rotoOmega  SampleTime=-1
      settings: Save2DSignal=2-D array (concatenate along first dimension)
  Transfer Fcn{,1..3} (4 alike) : TransferFcn  Commented=on  Denominator=[0.01 1]
  Transfer Fcn12 : TransferFcn  Commented=on  Denominator=[0.02 1]
  Vector Concatenate : Concatenate  Commented=on  NumInputs=4
  Vehicle Dynamics : Subsystem  Variant=on  VariantControlMode=label  LabelModeActiveChoice=Veh14DOF  mask{VehDynSel=Vehicle 14DOF}
      mask prompts: VehDynSel "Select the driver"
      mask init:
      | choice = get_param(gcb,'VehDynSel');
      | curBlk = gcb;
      | oldVariant = get_param(gcb,'LabelModeActiveChoice');
      | switch choice
      |     case 'Vehicle Longitudinal'
      |         set_param(curBlk, 'LabelModeActiveChoice', 'VehLong');
      | %     case 'Vehicle 3DOF'   
      | %         set_param(curBlk, 'LabelModeActiveChoice', 'Veh3DOF');
      |     case 'Vehicle 7DOF'   
      |         set_param(curBlk, 'LabelModeActiveChoice', 'Veh7DOF');
      |     case 'Vehicle 14DOF'   
      |         set_param(curBlk, 'LabelModeActiveChoice', 'Veh14DOF');
      | end
      mask TypeOptions VehDynSel: Vehicle Longitudinal | Vehicle 7DOF | Vehicle 14DOF
  VehicleSimulationType : Constant  Value=0
  omega : Scope
  Veh : Outport
  ManSpdSel : Outport  Port=2
  RototestInput : Outport  Port=3
  wires:
  "Powertrain Supervisory Controller "/1(SupvsryCtrl) -> Vehicle Dynamics/2(SupvsryCtrl), Motor/1(SupvsryCtrl), [SupvsryCtrl]
  Driver/1 -> "Powertrain Supervisory Controller "/1(Driver)
  Bus Creator/1 -> Veh/1  "Veh"
  [SupvsryCtrl] -> Bus Creator/1  "SupvsryCtrl"
  [Batt] -> Bus Creator/2  "Batt"
  [Mtr] -> Bus Creator/3  "Mtr"
  [Whl] -> Bus Creator/5  "Whl"
  [Chassis] -> Bus Creator/6  "Chassis"
  Battery/1(Batt) -> [Batt], "Powertrain Supervisory Controller "/4(Batt)
  Motor/1(Mtr) -> "Powertrain Supervisory Controller "/3(Mtr), [Mtr]
  Env/1 -> Vehicle Dynamics/1(Env)
  Vehicle Dynamics/2(Chassis) -> "Powertrain Supervisory Controller "/2(Chassis), [Chassis]
  Vehicle Dynamics/1(Whl) -> [Whl]
  [Whl] -> Bus Selector/1
  [Diff] -> Bus Creator/4  "Diff"
  Front Wheel Drive/1(Diff) -> [Diff]
  Front Wheel Drive/3(PropShaftSpd) -> MtT1/1, Motor/2(MtrSpd)
  Motor/2(MtrTrq) -> Front Wheel Drive/1(DrvShfTrq), MtT/1, [MtrTrq]
  Front Wheel Drive/2(AxlTrq) -> AxT/1, Vehicle Dynamics/3(AxlTrq)
  Rototest and ORNL Interface/2(Powertrain Out) -> Bus Selector3/1, Terminator/1
  Rototest and ORNL Interface/4(WhlSpd) -> To Workspace2/1, Terminator4/1  "WhlSpdCmd"
  Vehicle Dynamics/3(RototestInput) -> RototestInput/1, Goto6/1
  VehicleSimulationType/1 -> Multiport Switch/1
  Driver and Drive Cycle/1(DriverBus) -> Actuation and Outputs/1(Driver Commands)
  Bus Selector1/1 -> Data Type Conversion1/1  "<BRAKE_LAMP_BOOL_CAN>"
  Data Type Conversion/1 -> Goto8/1  "SteerAngleCAN"
  "Rototest UDP RX ExternalMode  "/1(Data Vector) -> Rototest and ORNL Interface/2(UDP Input)
  Data Type Conversion1/1 -> Rototest and ORNL Interface/3(BRAKE_PRESSED), Goto7/1, Terminator2/1  "BrakePressed_flag"
  Bus Selector1/2 -> Data Type Conversion/1  "<STEERING_ANGLE_DEG_CAN>"
  From CAN/1(IO_Out) -> Bus Selector1/1
  Actuation and Outputs/1(BrakeSwitch) -> From CAN/1(BrakeSwitch)
  Actuation and Outputs/2(CAVE_Driver) -> Terminator3/1  "CAVE_Driver_Cmd"
  Rototest and ORNL Interface/3(DataSend) -> "Rototest UDP TX ExternalMode  "/1(Rototest_UDP_TX)  "Rototest_UDP_TX"
  Rototest and ORNL Interface/1(BrakeUpd) -> Terminator1/1
  From7/1 -> Bus Selector2/1
  Bus Selector2/3 -> Rototest and ORNL Interface/5(FXIN)  "<Fx>"
  Bus Selector2/2 -> Transfer Fcn12/1  "<VehSpd>"
  Bus Selector2/1 -> Rototest and ORNL Interface/1(CarTrqT2W)  "<CarTrqT2W>"
  Bus Selector/1 -> Multiport Switch/2  "<Omega>"
  Bus Selector3/1 -> Transfer Fcn/1  "<PT IF WFL rotv>"
  Bus Selector3/2 -> Transfer Fcn1/1  "<PT IF WFR rotv>"
  Bus Selector3/3 -> Transfer Fcn2/1  "<PT IF WRL rotv>"
  Bus Selector3/4 -> Transfer Fcn3/1  "<PT IF WRR rotv>"
  Vector Concatenate/1 -> Scope/1, To Workspace1/1, Goto9/1
  [OmegaRoto] -> Multiport Switch/3
  Gain1/1 -> AxT2/1, Rototest and ORNL Interface/4(vehSpeedKph), Goto10/1  "VehSpdKph"
  Gain/1 -> Driver and Drive Cycle/1(Veh speed feedback [kph])
  DriveCycle_trigger/1 -> Driver and Drive Cycle/2(Veh speed cycle trigger)
  Multiport Switch/1 -> Front Wheel Drive/2(Omega), omega/1
  Constant/1 -> Switch/3
  Switch/1 -> Gain1/1
  Abs/1 -> Switch/2
  Transfer Fcn/1 -> Vector Concatenate/1
  Transfer Fcn1/1 -> Vector Concatenate/2
  Transfer Fcn2/1 -> Vector Concatenate/3
  Transfer Fcn3/1 -> Vector Concatenate/4
  Transfer Fcn12/1 -> Switch/1, Abs/1
  CarCmd/1 -> Actuation and Outputs/2(CarlaGBS), Driver and Drive Cycle/4(CarlaRef)
  Driver and Drive Cycle/2(ManSpdSel) -> ManSpdSel/1
  SUMO_speed_level/1 -> Driver and Drive Cycle/3(SUMO Veh speed Cmd Level)
  From8/1 -> Gain/1
  connections:
  Battery/RConn1 -- Motor/LConn1
